simulink model "prelab2_simulink_q2"  (R2017a)
settings: Solver=ode45  StartTime=0.0  StopTime=3.0  MaxStep=.001  RelTol=1e-3
values from neighbouring files (symbols this model uses):
  a = 0.5    [lab2.m]    (also in lab2_q2.m = -10)
  zeta = 2    [lab2.m]    (also in lab2_q2.m = 0.6)
settings Model: Creator=kg3  LastModifiedBy=kg3

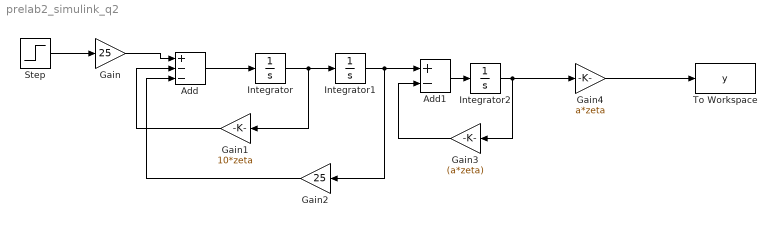
== system prelab2_simulink_q2 ==
  Add : Sum  Inputs=+--
  Add1 : Sum  Inputs=+-
  Gain : Gain  Gain=25
  Gain1 : Gain  Gain=10*zeta
  Gain2 : Gain  Gain=25
  Gain3 : Gain  Gain=(a*zeta)
  Gain4 : Gain  Gain=a*zeta
  Integrator : Integrator
  Integrator1 : Integrator
  Integrator2 : Integrator
  Step : Step  Time=0  SampleTime=0
  To Workspace : ToWorkspace  VariableName=y  SampleTime=-1
  wires:
  Step/1 -> Gain/1
  Integrator/1 -> Gain1/1, Integrator1/1
  Add/1 -> Integrator/1
  Gain/1 -> Add/1
  Gain1/1 -> Add/2
  Gain2/1 -> Add/3
  Integrator1/1 -> Add1/1, Gain2/1
  Integrator2/1 -> Gain4/1, Gain3/1
  Add1/1 -> Integrator2/1
  Gain3/1 -> Add1/2
  Gain4/1 -> To Workspace/1
